simulink model "blank_update"  (R2016b)
settings: Solver=ode1  StartTime=0.0  StopTime=10.0  FixedStep=0.001  RelTol=1e-3
libraries: simulink x9, quarc_library x4
settings Model: Creator=Ramin_hp  LastModifiedBy=Ramin_hp

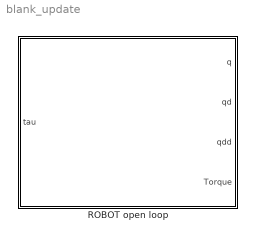
== system blank_update ==
  ROBOT open loop : Subsystem

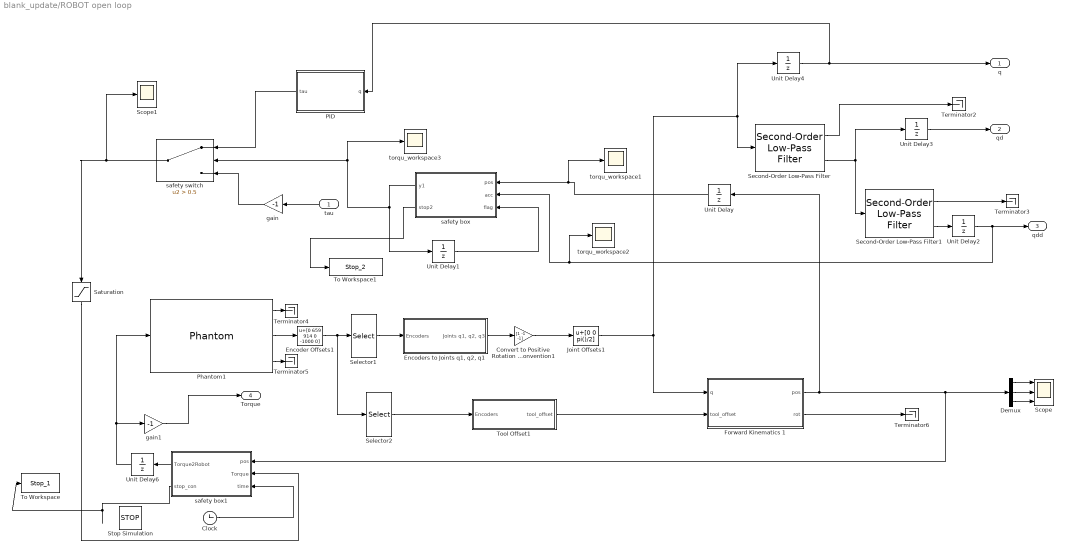
== system blank_update/ROBOT open loop ==
  tau : Inport
  Clock : Clock
  Convert to Positive Rotation Convention1 : Gain  Gain=[1 -1 -1]
  Demux : Demux  Outputs=3
  Encoder Offsets1 : Bias  Bias=[0 659 914 0 -1000 0]
  "Encoders to Joints q1, q2, q1" : Subsystem
  Forward Kinematics 1 : MATLAB Function  TreatAsAtomicUnit=on
  Joint Offsets1 : Bias  Bias=[0 0 pi()/2]
  PID : Subsystem
  Phantom1 : quarc_library/Devices/Third-Party/SensAble/Phantom/Phantom  device_name=Default Device  output_type=Encoders Values  input_type=Joint space  velocity_limit_option=on  velocity_limit=1200  is_7dof=off  sample_time=-1
      settings: AttributesFormatString=(%<device_name>)
  Saturation : Saturate  UpperLimit=0.3  LowerLimit=-0.3
  Scope : Scope  NumInputPorts=3
  Scope1 : Scope
  Second-Order Low-Pass Filter : quarc_library/Continuous/Second-Order Low-Pass Filter  params_source=Internal (dialog parameters)  input_width=10  input_zeta=1  input_init=0
  Second-Order Low-Pass Filter1 : quarc_library/Continuous/Second-Order Low-Pass Filter  params_source=Internal (dialog parameters)  input_width=10  input_zeta=1  input_init=0
  Selector1 : Selector  InputPortWidth=6  IndexOptions=Index vector (dialog)  Indices=[1:3]  OutputSizes=1
  Selector2 : Selector  InputPortWidth=6  IndexOptions=Index vector (dialog)  Indices=[4:6]  OutputSizes=1
  Stop Simulation : Stop
  Terminator{2..6} (5 alike) : Terminator
  To Workspace : ToWorkspace  VariableName=Stop_1  SampleTime=-1
  To Workspace1 : ToWorkspace  VariableName=Stop_2  SampleTime=-1
  Tool Offset1 : MATLAB Function  TreatAsAtomicUnit=on
  Unit Delay : UnitDelay  InitialCondition=[0.1 0 0]'  SampleTime=-1
  Unit Delay{1..4,6} (5 alike) : UnitDelay  SampleTime=-1
  gain : Gain  Gain=-1
  gain1 : Gain  Gain=-1
  safety box : MATLAB Function  TreatAsAtomicUnit=on
  safety box1 : MATLAB Function  TreatAsAtomicUnit=on
  safety switch : Switch  Criteria=u2 > Threshold  Threshold=0.5  SampleTime=1e-3
  torqu_workspace1 : Scope
  torqu_workspace2 : Scope
  torqu_workspace3 : Scope
  q : Outport
  qd : Outport  Port=2
  qdd : Outport  Port=3
  Torque : Outport  Port=4
  wires:
  Second-Order Low-Pass Filter/1 -> Terminator2/1
  Second-Order Low-Pass Filter1/1 -> Terminator3/1
  Second-Order Low-Pass Filter/2 -> Unit Delay3/1, Second-Order Low-Pass Filter1/1
  Convert to Positive Rotation Convention1/1 -> Joint Offsets1/1
  Phantom1/2 -> Encoder Offsets1/1
  Phantom1/3 -> Terminator5/1
  Phantom1/1 -> Terminator4/1
  Selector1/1 -> "Encoders to Joints q1, q2, q1"/1(Encoders)
  Encoder Offsets1/1 -> Selector2/1, Selector1/1
  "Encoders to Joints q1, q2, q1"/1("Joints q1, q2, q3") -> Convert to Positive Rotation Convention1/1
  Joint Offsets1/1 -> Unit Delay4/1, Second-Order Low-Pass Filter/1, Forward Kinematics 1/1(q)
  Forward Kinematics 1/2(rot) -> Terminator6/1
  Selector2/1 -> Tool Offset1/1(Encoders)
  Tool Offset1/1(tool_offset) -> Forward Kinematics 1/2(tool_offset)
  Demux/1 -> Scope/1
  Demux/2 -> Scope/2
  Demux/3 -> Scope/3
  tau/1 -> gain/1
  gain/1 -> safety switch/3
  safety box/1(y1) -> torqu_workspace3/1, safety switch/2, Unit Delay1/1
  safety switch/1 -> Scope1/1, Saturation/1
  Unit Delay/1 -> torqu_workspace1/1, safety box/1(pos)
  Unit Delay1/1 -> safety box/3(flag)
  Second-Order Low-Pass Filter1/2 -> Unit Delay2/1
  Unit Delay2/1 -> torqu_workspace2/1, safety box/2(acc), qdd/1
  Unit Delay3/1 -> qd/1
  Unit Delay4/1 -> PID/1(q), q/1
  PID/1(tau) -> safety switch/1
  Clock/1 -> safety box1/3(time)
  safety box1/1(Torque2Robot) -> Unit Delay6/1
  safety box1/2(stop_con) -> To Workspace/1
  Forward Kinematics 1/1(pos) -> Unit Delay/1, safety box1/1(pos), Demux/1
  Unit Delay6/1 -> Phantom1/1, gain1/1
  gain1/1 -> Torque/1
  Saturation/1 -> safety box1/2(Torque)
  safety box/2(stop2) -> To Workspace1/1

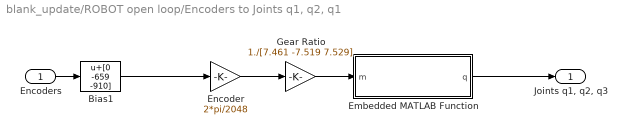
== system blank_update/ROBOT open loop/Encoders to Joints q1, q2, q1 ==
  Encoders : Inport
  Bias1 : Bias  Bias=[0 -659 -910]
  Embedded MATLAB Function : MATLAB Function  TreatAsAtomicUnit=on
  Encoder : Gain  Gain=2*pi/2048
  Gear Ratio : Gain  Gain=1./[7.461 -7.519 7.529]
  "Joints q1, q2, q3" : Outport
  wires:
  Embedded MATLAB Function/1(q) -> "Joints q1, q2, q3"/1
  Encoders/1 -> Bias1/1
  Encoder/1 -> Gear Ratio/1
  Gear Ratio/1 -> Embedded MATLAB Function/1(m)
  Bias1/1 -> Encoder/1

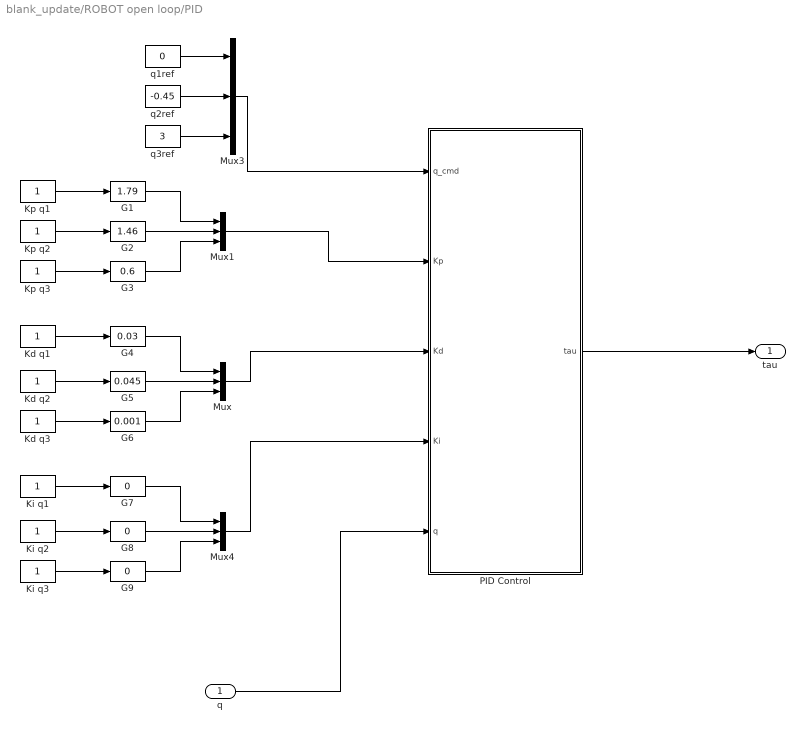
== system blank_update/ROBOT open loop/PID ==
  q : Inport
  G1 : simulink/Math Operations/Slider Gain  low=0  gain=1.79  high=2
  G2 : simulink/Math Operations/Slider Gain  low=0  gain=1.46  high=2
  G3 : simulink/Math Operations/Slider Gain  low=0  gain=0.6  high=1
  G4 : simulink/Math Operations/Slider Gain  low=0.02  gain=0.03  high=0.1
  G5 : simulink/Math Operations/Slider Gain  low=0.02  gain=0.045  high=0.1
  G6 : simulink/Math Operations/Slider Gain  low=0  gain=0.001  high=0.025
  G7 : simulink/Math Operations/Slider Gain  low=0  gain=0  high=2
  G8 : simulink/Math Operations/Slider Gain  low=0  gain=0  high=2
  G9 : simulink/Math Operations/Slider Gain  low=0  gain=0  high=3
  Kd q1 : Constant
  Kd q2 : Constant
  Kd q3 : Constant
  Ki q1 : Constant
  Ki q2 : Constant
  Ki q3 : Constant
  Kp q1 : Constant
  Kp q2 : Constant
  Kp q3 : Constant
  Mux{,1,3..4} (4 alike) : Mux  Inputs=3
  PID Control : Subsystem
  q1ref : Constant  Value=0
  q2ref : Constant  Value=-0.45
  q3ref : Constant  Value=3
  tau : Outport
  wires:
  Mux3/1 -> PID Control/1(q_cmd)
  Mux/1 -> PID Control/3(Kd)
  Mux1/1 -> PID Control/2(Kp)
  Kp q1/1 -> G1/1
  Kp q2/1 -> G2/1
  Kp q3/1 -> G3/1
  Kd q1/1 -> G4/1
  Kd q2/1 -> G5/1
  Kd q3/1 -> G6/1
  G1/1 -> Mux1/1
  G2/1 -> Mux1/2
  G3/1 -> Mux1/3
  G4/1 -> Mux/1
  G5/1 -> Mux/2
  G6/1 -> Mux/3
  Ki q1/1 -> G7/1
  Ki q2/1 -> G8/1
  Ki q3/1 -> G9/1
  G7/1 -> Mux4/1
  G8/1 -> Mux4/2
  G9/1 -> Mux4/3
  Mux4/1 -> PID Control/4(Ki)
  PID Control/1(tau) -> tau/1
  q/1 -> PID Control/5(q)
  q1ref/1 -> Mux3/1
  q2ref/1 -> Mux3/2
  q3ref/1 -> Mux3/3

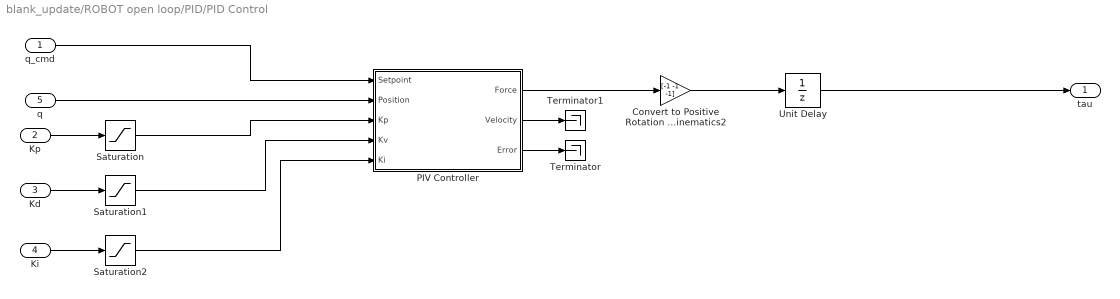
== system blank_update/ROBOT open loop/PID/PID Control ==
  q_cmd : Inport
  Kp : Inport  Port=2
  Kd : Inport  Port=3
  Ki : Inport  Port=4
  q : Inport  Port=5
  Convert to Positive Rotation Convension Used in Kinematics2 : Gain  Gain=[-1 -1 -1]
  PIV Controller : Subsystem
  Saturation : Saturate  UpperLimit=[2 2 1]  LowerLimit=[0 0 0]
  Saturation1 : Saturate  UpperLimit=[.1 .1 .025]  LowerLimit=[.02 .02 0]
  Saturation2 : Saturate  UpperLimit=[2 2 3]  LowerLimit=[0 0 0]
  Terminator : Terminator
  Terminator1 : Terminator
  Unit Delay : UnitDelay  SampleTime=-1
  tau : Outport
  wires:
  Saturation2/1 -> PIV Controller/5(Ki)
  Ki/1 -> Saturation2/1
  Saturation1/1 -> PIV Controller/4(Kv)
  Kd/1 -> Saturation1/1
  Saturation/1 -> PIV Controller/3(Kp)
  Kp/1 -> Saturation/1
  q_cmd/1 -> PIV Controller/1(Setpoint)
  PIV Controller/2(Velocity) -> Terminator1/1
  PIV Controller/3(Error) -> Terminator/1
  PIV Controller/1(Force) -> Convert to Positive Rotation Convension Used in Kinematics2/1
  Convert to Positive Rotation Convension Used in Kinematics2/1 -> Unit Delay/1
  Unit Delay/1 -> tau/1
  q/1 -> PIV Controller/2(Position)

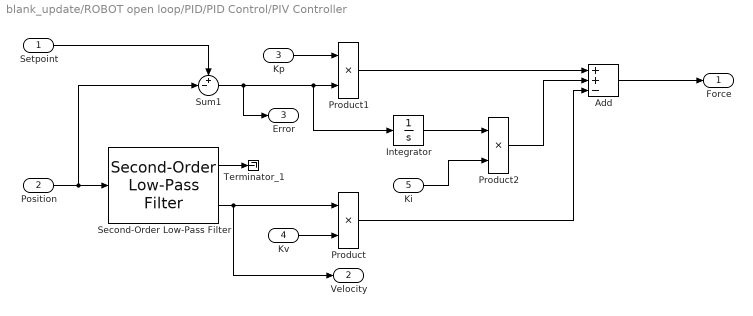
== system blank_update/ROBOT open loop/PID/PID Control/PIV Controller ==
  Setpoint : Inport
  Position : Inport  Port=2
  Kp : Inport  Port=3
  Kv : Inport  Port=4
  Ki : Inport  Port=5
  Add : Sum  Inputs=++-
  Integrator : Integrator
  Product : Product  RndMeth=Zero
  Product1 : Product  RndMeth=Zero
  Product2 : Product  RndMeth=Zero
  Second-Order Low-Pass Filter : quarc_library/Continuous/Second-Order Low-Pass Filter  params_source=Internal (dialog parameters)  input_width=200  input_zeta=1  input_init=0
  Sum1 : Sum  Inputs=+-|
  Terminator_1 : Terminator
  Force : Outport
  Velocity : Outport  Port=2
  Error : Outport  Port=3
  wires:
  Position/1 -> Sum1/2, Second-Order Low-Pass Filter/1
  Second-Order Low-Pass Filter/2 -> Velocity/1, Product/1
  Kp/1 -> Product1/1
  Setpoint/1 -> Sum1/1
  Sum1/1 -> Error/1, Product1/2, Integrator/1
  Kv/1 -> Product/2
  Second-Order Low-Pass Filter/1 -> Terminator_1/1
  Integrator/1 -> Product2/1
  Ki/1 -> Product2/2
  Product1/1 -> Add/1
  Product2/1 -> Add/2
  Product/1 -> Add/3
  Add/1 -> Force/1

== matlab function blank_update/ROBOT open loop/safety box1 ==
  data: pos input; Torque input; Torque2Robot output; time input; stop_con output
function [Torque2Robot,stop_con] = fcn(pos,Torque,time)

% gives 0 input torque if x,y,z are out of the safety box or the max
% acceleration is exceeded
stop_con=0;

x=pos(1);
y=pos(2);
z=pos(3);

xmin = 0.16-0.01;
xmax = 0.16+0.01;
ymin = 0-0.01;
ymax = 0+0.01;
zmin = -0.13-0.01;
zmax = -0.13+0.01;

if (time<0.002)
    if x<xmin || x>xmax || y<ymin || y>ymax || z<zmin || z>zmax
        stop_con=1;
    end
end

Torque2Robot = Torque;

== matlab function blank_update/ROBOT open loop/Encoders to Joints q1, q2, q1/Embedded MATLAB Function ==
  data: m input; q output
function q = Motors_2_Joints(m)
q = m;
q(1) = m(1);
q(2) = m(2);
q(3) = m(3) - m(2) -pi/2;
end

== matlab function blank_update/ROBOT open loop/Forward Kinematics 1 ==
  data: pos output; q input; rot output; tool_offset input
function [pos,rot]    = ForwardKinematics(q,tool_offset)
% This block supports the Embedded MATLAB subset.
% See the help menu for details. 

% Link lengths
L1 = .132;
L2 = .132;

%Define A-matrices
%A1= DH(theta ,d ,a ,alpha)
A1 = DH(q(1), 0, 0, -pi()/2);
A2 = DH(q(2), 0, L1, 0);
A3 = DH(q(3)-pi/2, 0, L2, 0);

%Define T Matrices
T01=A1;
T02=T01*A2;
T03=T02*A3;

%tool_offset given with respect to frame 3.
T_tool=T03*tool_offset;
rot=T_tool(1:3,1:3);
pos=T_tool(1:3,4);

%Axes of rotation in base coordinates. 
z0=[0 0 1]';
z1=T01(1:3,3);
z2=T02(1:3,3);

%Coordinate Frame origins in Base frame coordinates
p0=[0 0 0]';
p1=T01(1:3,4);
p2=T02(1:3,4);
p3=T03(1:3,4);

%Formulation of the Jacobian

%%%%%%%%%%%%%%%%%%%%%%%%%%%%%%%%%%%%%%%%%%%%%%%%%%%%
%jac = [cross(z0,(pos-p0)) cross(z1,(pos-p1)) cross(z2,(pos-p2))
 %   z0 z1 z2];

end

function A = DH(theta, d, a, alpha)

A_R_z = [cos(theta) -sin(theta) 0 0;
         sin(theta) cos(theta) 0 0;
         0 0 1 0;
         0 0 0 1];

A_T_z = [1 0 0 0;
         0 1 0 0;
         0 0 1 d;
         0 0 0 1];
     
  

A_T_x = [1 0 0 a;
         0 1 0 0;
         0 0 1 0;
         0 0 0 1];

A_R_x = [1 0 0 0;
         0 cos(alpha) -sin(alpha)  0;
         0 sin(alpha) cos(alpha) 0;
         0 0 0 1];

A = A_R_z*A_T_z*A_T_x*A_R_x;

end

== matlab function blank_update/ROBOT open loop/Tool Offset1 ==
  data: Encoders input; tool_offset output
function tool_offset = getToolOffset(Encoders)

%convert encoder values to angles using bias and gain
bias = [-2048 -2654 -2048];
gain = [2*pi()/4915 2*pi()/4096 2*pi()/4915];
Angle = (Encoders' + bias).*gain;

% convert the angle to the positive rotation convention defined
% by DH parameters
pos_rot = [-1 1 1];
joint_offset = [0 -(40-180)*pi/180 0];
Joint456 = Angle.*pos_rot + joint_offset;

%pick off theta4 and theta5
theta4 = Joint456(1);
theta5 = Joint456(2);

% The orientation of the tool offset matrix is given two successive
% rotations about x and z axis. 
RotZ = [cos(theta5) -sin(theta5) 0; sin(theta5) cos(theta5) 0; 0 0 1];
RotX = [1 0 0; 0 cos(theta4) -sin(theta4); 0 sin(theta4) cos(theta4)];
R = RotX*RotZ; % R is the rotation matrix of the tool offset matrix with respect to frame 3

% with respect to frame 3, the tool is 0.039m in the x-direction. Convert
% this vector to tool frame coordinates
tool_pos =R * [.039; 0; 0];

%create a Tool_offset transformation matrix. Use Identity matrix for
%rotation to show that the end effector frame and frame 3 are always
%aligned
I = [1 0 0; 0 1 0; 0 0 1];
tool = cat(2,I,tool_pos);
tool_offset = cat(1,tool,[0 0 0 1]);

== matlab function blank_update/ROBOT open loop/safety box ==
  data: pos input; acc input; y1 output; flag input; stop2 output
function [y1,stop2] = fcn(pos,acc,flag)

% gives 0 input torque if x,y,z are out of the safety box or the max
% acceleration is exceeded

stop2 = 0;

x=pos(1);
y=pos(2);
z=pos(3);

% xmin = -0.22;
% xmax = 0.22;
% ymin = -0.1;
% ymax = 0.1;
% zmin = -0.14;
% zmax = 0.04;
xmin = 0.05;
xmax = 0.3;
ymin = -0.13;
ymax = 0.13;
zmin = -0.14;
zmax = 0.05;

acc1 = abs(acc(1));
acc2 = abs(acc(2));
acc3 = abs(acc(3));
acc_max = [30; 30; 60];

if flag==0
    if x<xmin || x>xmax || y<ymin || y>ymax || z<zmin || z>zmax || acc1>acc_max(1) || acc2>acc_max(2) || acc3>acc_max(3)
        flag=1;
        stop2 = 1;
    end
end

y1 = flag;
